simulink model "VectorMode"  (R2018a)
settings: Solver=VariableStepAuto  StartTime=0.0  StopTime=30  RelTol=1e-3
libraries: dspmtrx3 x2, NetworkEmulator x1
settings Model: Creator=mostafa  LastModifiedBy=mostafa

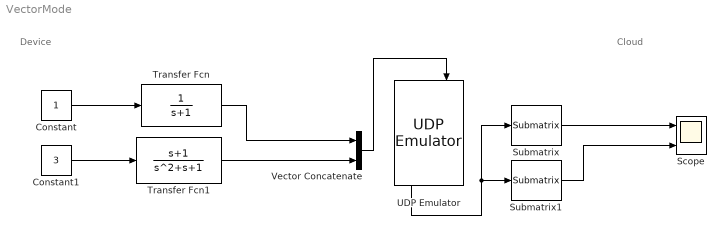
== system VectorMode ==
  note: Cloud
  note: Device
  Constant : Constant
  Constant1 : Constant  Value=3
  Scope : Scope  NumInputPorts=2
  Submatrix : dspmtrx3/Submatrix  RowSpan=One row  RowStartMode=Index  RowStartIndex=1  RowEndMode=Last  RowEndIndex=1  ColSpan=One column  ColStartMode=Index  ColStartIndex=1  ColEndMode=Last  ColEndIndex=1
  Submatrix1 : dspmtrx3/Submatrix  RowSpan=One row  RowStartMode=Index  RowStartIndex=2  RowEndMode=Last  RowEndIndex=1  ColSpan=One column  ColStartMode=Index  ColStartIndex=1  ColEndMode=Last  ColEndIndex=1
  Transfer Fcn : TransferFcn  Denominator=[1 1]
  Transfer Fcn1 : TransferFcn  Numerator=[1 1]  Denominator=[1 1 1]
  UDP Emulator : NetworkEmulator/UDP Emulator  CloudSampleInterval=500  DeviceSampleInterval=500  MeanDelay=100  Jitter=10  LossModel=Independent Random  Loss=0  P_loss=0  E_B=5  rho=99  P_isol=0  E_GB=2
  Vector Concatenate : Concatenate
  wires:
  Constant/1 -> Transfer Fcn/1
  Constant1/1 -> Transfer Fcn1/1
  Transfer Fcn/1 -> Vector Concatenate/1
  Transfer Fcn1/1 -> Vector Concatenate/2
  Submatrix1/1 -> Scope/2
  Submatrix/1 -> Scope/1
  UDP Emulator/1 -> Submatrix1/1, Submatrix/1
  Vector Concatenate/1 -> UDP Emulator/2
